simulink model "host_model"  (R2023b)
settings: Solver=FixedStepDiscrete  StartTime=0.0  StopTime=Inf  RelTol=1e-3  EnableMultiTasking=on
values from neighbouring files (symbols this model uses):
  n = 500    [init_hw.m]    (also in init_psc_hw.m = 300)
  T_s = 1/(2*f_sw)    (= 0.0001)    [init_hw.m]    (also in init_psc_hw.m)
libraries: instrumentseriallib x3
settings Model: Creator=maatt  LastModifiedBy=maatt
settings DataIOCC: SaveOutput=off  DSMLogging=off  InspectSignalLogs=on  SaveTime=off  ReturnWorkspaceOutputs=off

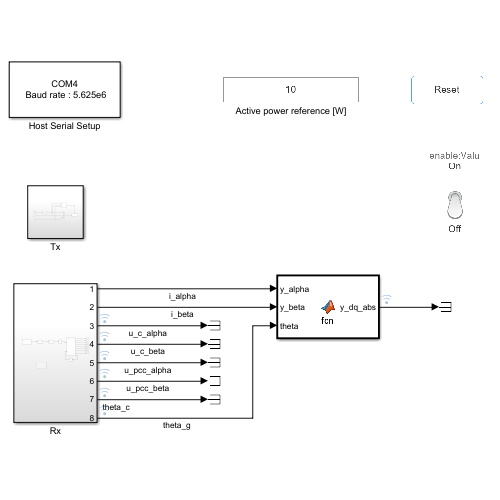
[thumbnail: Simulink's stored preview of the top-level diagram]
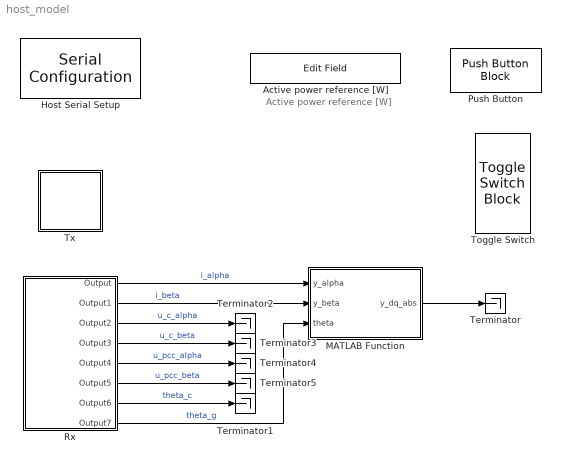
== system host_model ==
  note: Active power reference [W]
  Active power reference [W] : EditField  LabelPosition=Hide  ShowInitialText=on  Alignment=Center
  Host Serial Setup : instrumentseriallib/Serial Configuration  Priority=-99  PortSel=COM4  Port=COM4  ComPort=COM4  BaudRate=5.625e6  DataBits=8  Parity=none  StopBits=1  ByteOrder=little-endian  FlowControl=none  Timeout=2  SimulateUsing=Interpreted execution  BlockInModel=on  aMode=5
      settings: LibrarySourceBlock=mcblib/Protection and Diagnostics/Host Serial Setup
  MATLAB Function : MATLAB Function  TreatAsAtomicUnit=on
  Push Button : PushButtonBlock  ButtonText=Reset  OffValue=0.000000
  Rx : Subsystem
  Terminator{,1..5} (6 alike) : Terminator
  Toggle Switch : ToggleSwitchBlock
      settings: Values={{'Off', 'On'}, [0 1]}
  Tx : Subsystem
  wires:
  Rx/1(Output) -> MATLAB Function/1(y_alpha)  "i_alpha"
  Rx/2(Output1) -> MATLAB Function/2(y_beta)  "i_beta"
  Rx/3(Output2) -> Terminator2/1  "u_c_alpha"
  Rx/4(Output3) -> Terminator3/1  "u_c_beta"
  Rx/5(Output4) -> Terminator4/1  "u_pcc_alpha"
  Rx/6(Output5) -> Terminator5/1  "u_pcc_beta"
  Rx/8(Output7) -> MATLAB Function/3(theta)  "theta_g"
  MATLAB Function/1(y_dq_abs) -> Terminator/1
  Rx/7(Output6) -> Terminator1/1  "theta_c"

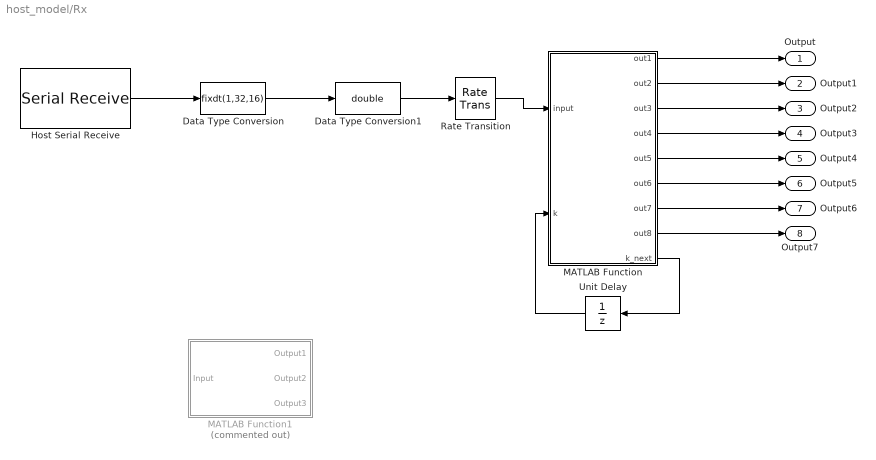
== system host_model/Rx ==
  Data Type Conversion : DataTypeConversion  OutDataTypeStr=fixdt(1,32,16)  ConvertRealWorld=Stored Integer (SI)  RndMeth=Simplest  SaturateOnIntegerOverflow=off
  Data Type Conversion1 : DataTypeConversion  OutDataTypeStr=double  RndMeth=Simplest  SaturateOnIntegerOverflow=off
  Host Serial Receive : instrumentseriallib/Serial Receive  PortSel=COM4  Port=COM4  ComPort=COM4  DataType=uint32  SaveDataType=uint8  ToggleHeader=on  Header='SSSS'  ToggleTerminator=on  Terminator=Custom terminator  CustomTerminator='EEEE'  InputFormat=Row major  ToggleDataSize=on  DataSize=[n 8]  EnableBlockingMode=on  ActionDataUnavailable=Output custom value  ActionWhenDataUnavailable=Output custom value  CustomValue=4  SampleTime=2*n*T_s  SimulateUsing=Interpreted execution  BlockInModel=on  aMode=5
      settings: LibrarySourceBlock=mcbhostblockslib/Host Serial Receive
  MATLAB Function : MATLAB Function  TreatAsAtomicUnit=on  SystemSampleTime=2*T_s
  MATLAB Function1 : MATLAB Function  Commented=on  TreatAsAtomicUnit=on
  Rate Transition : RateTransition  Deterministic=off  OutPortSampleTime=2*T_s
  Unit Delay : UnitDelay  InitialCondition=1  SampleTime=2*T_s  HasFrameUpgradeWarning=on
  Output : Outport
  Output1 : Outport  Port=2
  Output2 : Outport  Port=3
  Output3 : Outport  Port=4
  Output4 : Outport  Port=5
  Output5 : Outport  Port=6
  Output6 : Outport  Port=7
  Output7 : Outport  Port=8
  wires:
  Data Type Conversion/1 -> Data Type Conversion1/1
  Host Serial Receive/1 -> Data Type Conversion/1
  MATLAB Function/1(out1) -> Output/1
  MATLAB Function/2(out2) -> Output1/1
  MATLAB Function/3(out3) -> Output2/1
  Data Type Conversion1/1 -> Rate Transition/1
  Unit Delay/1 -> MATLAB Function/2(k)
  MATLAB Function/9(k_next) -> Unit Delay/1
  Rate Transition/1 -> MATLAB Function/1(input)
  MATLAB Function/4(out4) -> Output3/1
  MATLAB Function/5(out5) -> Output4/1
  MATLAB Function/6(out6) -> Output5/1
  MATLAB Function/7(out7) -> Output6/1
  MATLAB Function/8(out8) -> Output7/1

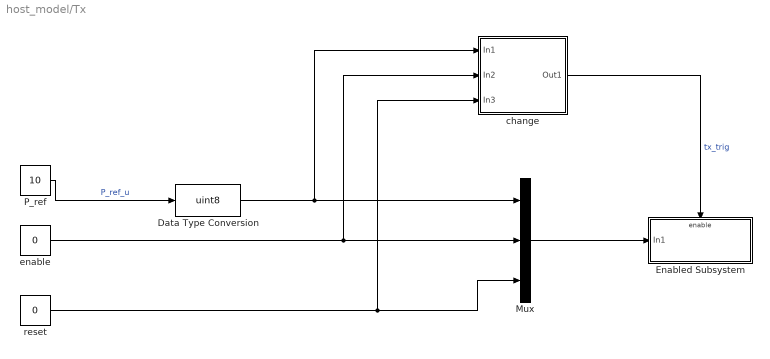
== system host_model/Tx ==
  Data Type Conversion : DataTypeConversion  OutDataTypeStr=uint8  RndMeth=Simplest  SaturateOnIntegerOverflow=off
  Enabled Subsystem : Subsystem  TreatAsAtomicUnit=on
  Mux : Mux  Inputs=3
  P_ref : Constant  Value=10  OutDataTypeStr=uint32  SampleTime=n*T_s
  change : Subsystem
  enable : Constant  Value=0  VectorParams1D=off  OutDataTypeStr=uint8  SampleTime=n*T_s
  reset : Constant  Value=0  VectorParams1D=off  OutDataTypeStr=uint8  SampleTime=n*T_s
  wires:
  reset/1 -> change/3(In3), Mux/3
  Mux/1 -> Enabled Subsystem/1(In1)
  change/1(Out1) -> Enabled Subsystem/Enable  "tx_trig"
  enable/1 -> change/2(In2), Mux/2
  P_ref/1 -> Data Type Conversion/1  "P_ref_u"
  Data Type Conversion/1 -> change/1(In1), Mux/1

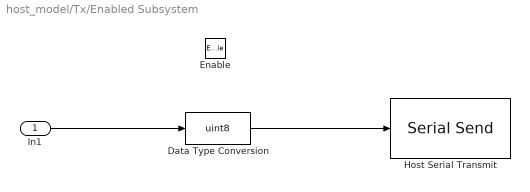
== system host_model/Tx/Enabled Subsystem ==
  In1 : Inport
  Enable : EnablePort
  Data Type Conversion : DataTypeConversion  OutDataTypeStr=uint8  RndMeth=Simplest  SaturateOnIntegerOverflow=off
  Host Serial Transmit : instrumentseriallib/Serial Send  PortSel=COM4  Port=COM4  ComPort=COM4  Header=[]  Terminator=<none>  CustomTerminator='E'  EnableBlockingMode=on  SimulateUsing=Interpreted execution  BlockInModel=on  aMode=5
      settings: LibrarySourceBlock=mcblib/Protection and Diagnostics/Host Serial Transmit
  wires:
  In1/1 -> Data Type Conversion/1
  Data Type Conversion/1 -> Host Serial Transmit/1

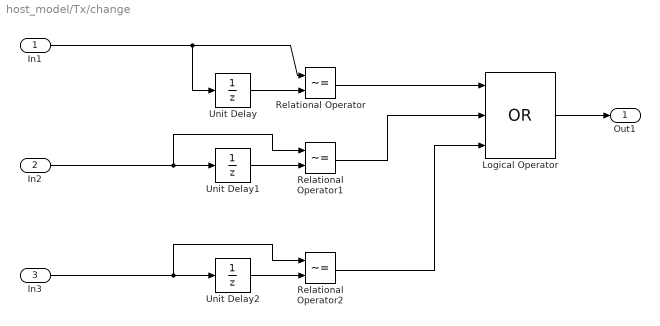
== system host_model/Tx/change ==
  In1 : Inport
  In2 : Inport  Port=2
  In3 : Inport  Port=3
  Logical Operator : Logic  Operator=OR  Inputs=3  AllPortsSameDT=off  OutDataTypeStr=boolean
  Relational Operator : RelationalOperator  Operator=~=  OutDataTypeStr=boolean  InputSameDT=off
  Relational Operator1 : RelationalOperator  Operator=~=  OutDataTypeStr=boolean  InputSameDT=off
  Relational Operator2 : RelationalOperator  Operator=~=  OutDataTypeStr=boolean  InputSameDT=off
  Unit Delay : UnitDelay  SampleTime=n*T_s  HasFrameUpgradeWarning=on
  Unit Delay1 : UnitDelay  SampleTime=n*T_s  HasFrameUpgradeWarning=on
  Unit Delay2 : UnitDelay  SampleTime=n*T_s  HasFrameUpgradeWarning=on
  Out1 : Outport  VectorParamsAs1DForOutWhenUnconnected=off
  wires:
  Unit Delay2/1 -> Relational Operator2/2
  Relational Operator2/1 -> Logical Operator/3
  In3/1 -> Unit Delay2/1, Relational Operator2/1
  Logical Operator/1 -> Out1/1
  Relational Operator/1 -> Logical Operator/1
  In1/1 -> Relational Operator/1, Unit Delay/1
  Unit Delay/1 -> Relational Operator/2
  Unit Delay1/1 -> Relational Operator1/2
  Relational Operator1/1 -> Logical Operator/2
  In2/1 -> Unit Delay1/1, Relational Operator1/1

== matlab function host_model/Rx/MATLAB Function1 ==
  data: Output1 output; Output2 output; Input input; Output3 output
function [ Output1, Output2, Output3] = unBuf(Input)

Output1= Input(:, 1);
Output2 = Input(:, 2);
Output3 = Input(:, 3);
end

== matlab function host_model/Rx/MATLAB Function ==
  data: input input; out1 output; out2 output; out3 output; out4 output; out5 output; out6 output; out7 output; out8 output; k input; n parameter; k_next output
function [out1, out2, out3, out4, out5, out6, out7, out8, k_next]  = fcn(input, k, n)

out1 = input(k, 1);
out2 = input(k, 2);
out3 = input(k, 3);
out4 = input(k, 4);
out5 = input(k, 5);
out6 = input(k, 6);
out7 = input(k, 7);
out8 = input(k, 8);

if(k>=n)
    k_next=1;
else
    k_next = k+1;
end

== matlab function host_model/MATLAB Function ==
  data: y_alpha input double; y_dq_abs output double; y_beta input double; theta input
function y_dq_abs = fcn(y_alpha, y_beta, theta)

% Coordinate Transformation (Alpha-beta to dq)
y_s = y_alpha + 1j*y_beta;
y_dq_abs = abs(y_s * exp(-1j*theta));
